simulink model "analogmotorlab_startingpoint_2015a"  (R2016b)
settings: Solver=ode23tb  StartTime=0.0  StopTime=3  RelTol=1e-9  EnableMultiTasking=on
values from neighbouring files (symbols this model uses):
  K_m = a*tau_m    (= 0.6)    [run_me.m]
  K_p = 1    [run_me.m]
  T_i = 0.1    [run_me.m]
  tau_m = 0.04    [run_me.m]
undefined symbols (not defined in the file or in its folder): tacho2pot, V_s
settings Model: Creator=klasbo  LastModifiedBy=rende_000
settings DataIOCC: LimitDataPoints=on
settings OptimizationCC: LifeSpan=inf
settings DebuggingCC: SFUnexpectedBacktrackingDiag=warning  SFNoUnconditionalDefaultTransitionDiag=warning  SFExecutionAtInitializationDiag=none
settings HardwareCC: ProdBitPerSizeT=32  ProdBitPerPtrDiffT=32  ProdWordSize=32  ProdHWDeviceType=Specified
settings ModelReferenceCC: PropagateSignalLabelsOutOfModel=off
settings GRTTargetCC: TargetLangStandard=C89/C90 (ANSI)
settings ConfigComp: CovMetricSettings=dw  CovHtmlReporting=on  CovSaveCumulativeToWorkspaceVar=on  CovSaveSingleToWorkspaceVar=on  CovExternalEMLEnable=off

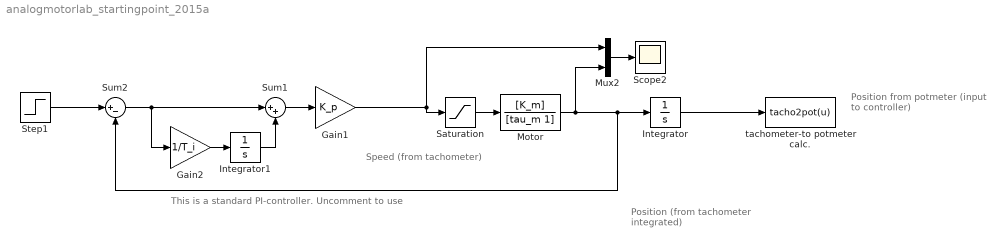
== system analogmotorlab_startingpoint_2015a ==
  note: Position from potmeter
      | (input to controller)
  note: Position
      | (from tachometer
      | integrated)
  note: Speed
      | (from tachometer)
  note: This is a standard PI-controller. Uncomment to use
  Gain1 : Gain  Gain=K_p
  Gain2 : Gain  Gain=1/T_i
  Integrator : Integrator
  Integrator1 : Integrator
  Motor : TransferFcn  Numerator=[K_m]  Denominator=[tau_m 1]
  Mux2 : Mux  Inputs=2
  Saturation : Saturate  UpperLimit=V_s  LowerLimit=-V_s
  Scope2 : Scope
  Step1 : Step  SampleTime=0
  Sum1 : Sum  Inputs=|++
  Sum2 : Sum  Inputs=|+-
  tachometer-to potmeter calc. : MATLABFcn  MATLABFcn=tacho2pot(u)
  wires:
  Saturation/1 -> Motor/1
  Motor/1 -> Mux2/2, Sum2/2, Integrator/1
  Integrator/1 -> tachometer-to potmeter calc./1
  Gain2/1 -> Integrator1/1
  Integrator1/1 -> Sum1/2
  Mux2/1 -> Scope2/1
  Sum1/1 -> Gain1/1
  Gain1/1 -> Saturation/1, Mux2/1
  Sum2/1 -> Gain2/1, Sum1/1
  Step1/1 -> Sum2/1
